simulink model "untitled"  (R2025b)
settings: Solver=VariableStepAuto  StartTime=0.0  StopTime=2  RelTol=1e-3
values from neighbouring files (symbols this model uses):
  b1 = 0.06    [definicje.m]
  J = 25e-3    (= 0.025)    [definicje.m]
  kfi = 1.4    [definicje.m]
  Ra = 3.0    (= 3)    [definicje.m]
  tau = La/Ra    (= 0.00333333333333)    [definicje.m]
  Ua = 100    [definicje.m]
settings Model: Creator=Student  LastModifiedBy=janek
settings ModelReferenceCC: EnableRefExpFcnMdlSchedulingChecks=on
settings RTWCC: GPUComputeCapability=3.5
settings SimscapeCC: SimscapeLogDataHistory=5000  SimscapeLogDecimation=1

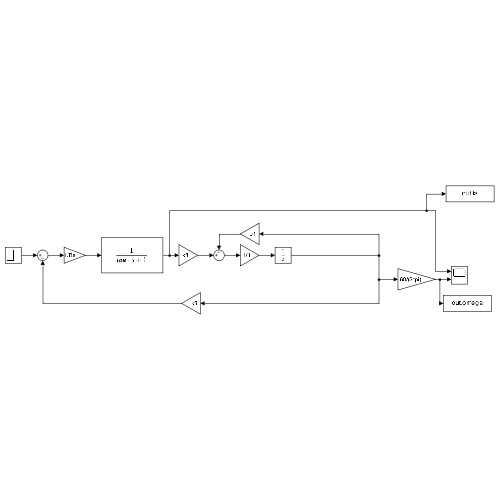
[thumbnail: Simulink's stored preview of the top-level diagram]
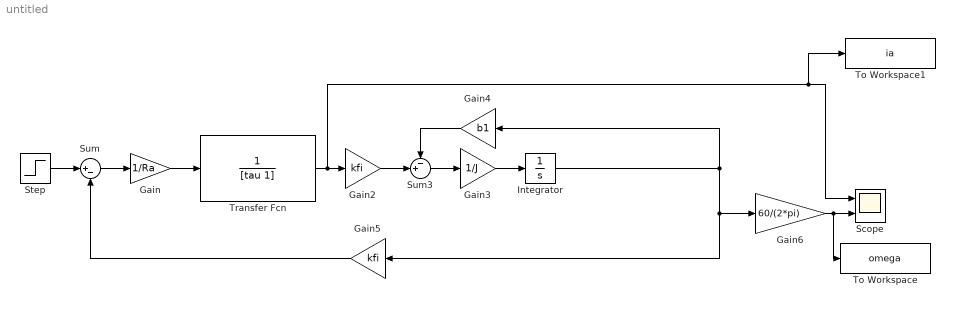
== system untitled ==
  Gain : Gain  Gain=1/Ra
  Gain2 : Gain  Gain=kfi
  Gain3 : Gain  Gain=1/J
  Gain4 : Gain  Gain=b1
  Gain5 : Gain  Gain=kfi
  Gain6 : Gain  Gain=60/(2*pi)
  Integrator : Integrator
  Scope : Scope  NumInputPorts=2
      settings: ActiveDisplayYMinimum=-7.7564072317620418  ActiveDisplayYMaximum=69.807665085858389
  Step : Step  After=Ua  SampleTime=0
  Sum : Sum  Inputs=|+-
  Sum3 : Sum  Inputs=-+|
  To Workspace : ToWorkspace  VariableName=omega  SaveFormat=Structure With Time  SampleTime=-1
  To Workspace1 : ToWorkspace  VariableName=ia  SaveFormat=Structure With Time  SampleTime=-1
  Transfer Fcn : TransferFcn  Denominator=[tau 1]
  wires:
  Sum/1 -> Gain/1
  Gain/1 -> Transfer Fcn/1
  Transfer Fcn/1 -> To Workspace1/1, Scope/1, Gain2/1
  Gain2/1 -> Sum3/2
  Sum3/1 -> Gain3/1
  Gain3/1 -> Integrator/1
  Integrator/1 -> Gain6/1, Gain5/1, Gain4/1
  Gain4/1 -> Sum3/1
  Gain5/1 -> Sum/2
  Step/1 -> Sum/1
  Gain6/1 -> To Workspace/1, Scope/2
